simulink model "test_asus"  (R2015a)
settings: Solver=ode3  StartTime=0.0  StopTime=5.0  RelTol=1e-3
values from neighbouring files (symbols this model uses):
  cx = 159.5    [Initialize_camera.m]
  cy = 119.5    [Initialize_camera.m]
  focal = 525/2    (= 262.5)    [Initialize_camera.m]
  interval = 5    [Initialize_camera.m]
settings Model: SimulationMode=external  ExtModeTrigDuration=100  Creator=sarag  LastModifiedBy=Amanda
settings OptimizationCC: OptimizeModelRefInitCode=on  LifeSpan=1  MaxStackSize=64
settings DebuggingCC: UnderspecifiedInitializationDetection=Classic  MergeDetectMultiDrivingBlocksExec=none
settings HardwareCC: ProdLargestAtomicInteger=Long  ProdLargestAtomicFloat=Double  ProdEndianess=LittleEndian  ProdHWDeviceType=ARM Compatible->ARM Cortex
settings RTWCC: SystemTargetFile=realtime.tlc  GenerateMakefile=off  TemplateMakefile=realtime.tmf  Description=Run on Target Hardware  RTWVerbose=off  Toolchain=Linaro Toolchain v4.8
settings ERTTargetCC: CombineOutputUpdateFcns=off  ExtModeMexArgs='192.168.7.2' 0 17725  ERTSrcFileBannerTemplate=realtime_code_template.cgt  ERTHdrFileBannerTemplate=realtime_code_template.cgt  ERTDataSrcFileTemplate=realtime_code_template.cgt  ERTDataHdrFileTemplate=realtime_code_template.cgt  ERTCustomFileTemplate=realtime_file_process.tlc

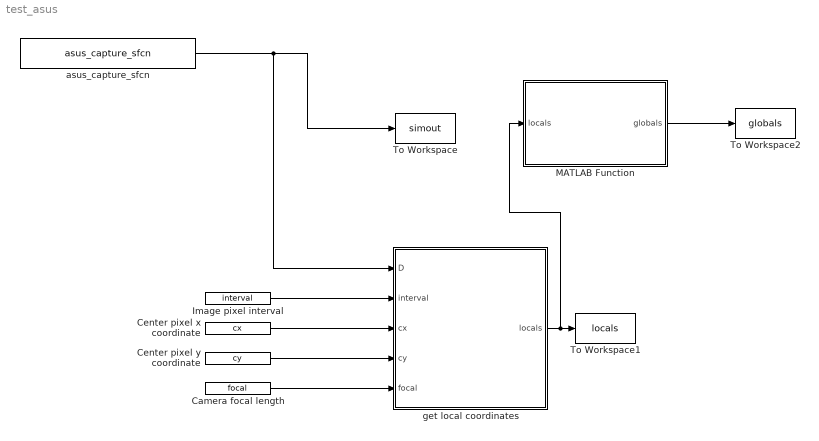
== system test_asus ==
  Camera focal length : Constant  Value=focal  SampleTime=-1
  Center pixel x coordinate : Constant  Value=cx  SampleTime=-1
  Center pixel y coordinate : Constant  Value=cy  SampleTime=-1
  Image pixel interval : Constant  Value=interval  SampleTime=-1
  MATLAB Function : MATLAB Function  TreatAsAtomicUnit=on
  To Workspace : ToWorkspace  VariableName=simout  SampleTime=-1
  To Workspace1 : ToWorkspace  VariableName=locals  SampleTime=-1
  To Workspace2 : ToWorkspace  VariableName=globals  SampleTime=-1
  asus_capture_sfcn : S-Function  FunctionName=asus_capture_sfcn  Parameters=SampleTime  mask(Legacy Function){SFunctionSpec=asusCapture(uint16 y1[240][320]), SampleTime=-1, ShowSpec=on}
      mask prompts: SampleTime "Sample time (-1 for inherited):"; ShowSpec "Display function specification"
      mask help:
      | This block allows you to call the legacy functions specified by the following Legacy Code Tool definition:
      | def.SFunctionName = 'asus_capture_sfcn';
      | def.OutputFcnSpec = 'asusCapture(uint16 y1[240][320])';
      | def.StartFcnSpec = 'asusInit()';
      | def.TerminateFcnSpec = 'asusTerminate()';
      | def.HeaderFiles = {'asus_capture.h', 'NI.h', 'wrapper.h'};
      | def.SourceFiles = {'wrapper.c'};
      | def.TargetLibFiles = {'libNI.so'};
      | def.IncPaths = {'.\include'};
      | def.SrcPaths = {'.\src'};
      | def.SampleTime = 'parameterized';
      | def.Options.isMacro = true;
      | def.Options.useTlcWithAccel = false;
      mask Help: <p>This block was generated automatically by the Legacy Code Tool. For detailed help on this tool, call<a href="matlab:legacy_code('help')"> legacy_code('help')</a>.</p>
      mask Callback ShowSpec:
      | if strcmp(get_param(gcbh, 'ShowSpec'), 'on')
      |   set_param(gcbh, 'MaskDisplay', sprintf('fprintf(''%s'');', get_param(gcbh, 'SFunctionSpec')));
      | else
      |   set_param(gcbh, 'MaskDisplay', sprintf('fprintf(''%s'');', get_param(gcbh, 'FunctionName')));
      | end
      mask Display: fprintf('asusCapture(uint16 y1[240][320])');
  get local coordinates : MATLAB Function  TreatAsAtomicUnit=on
  wires:
  Image pixel interval/1 -> get local coordinates/2(interval)
  Center pixel x coordinate/1 -> get local coordinates/3(cx)
  Center pixel y coordinate/1 -> get local coordinates/4(cy)
  Camera focal length/1 -> get local coordinates/5(focal)
  asus_capture_sfcn/1 -> get local coordinates/1(D), To Workspace/1
  get local coordinates/1(locals) -> MATLAB Function/1(locals), To Workspace1/1
  MATLAB Function/1(globals) -> To Workspace2/1

== matlab function test_asus/MATLAB Function ==
  data: locals input; globals output
function globals   = getGlobalCoordinates(locals)
B = zeros(size(locals));
Bt = zeros(4,length(locals));
globals = zeros(size(locals));


dt = zeros(4,4);

x = zeros(1, 3072);
y = zeros(1, 3072);
z = zeros(1, 3072);

R = eye(3);
    t = zeros(3,1);

    dt = [R t; 0 0 0 1];
    % Transformed cloud
    Bt = dt * [locals; ones(1,size(locals,2))];
    globals = Bt(1:3, :);  
    
end

== matlab function test_asus/get local coordinates ==
  data: D input; locals output; interval input; cx input; cy input; focal input
function locals = getLocalCoordinates(D, interval, cx,cy, focal)
%#codegen
a = 1;
x = zeros(1, 3072); %12288
y = zeros(1, 3072);
z = zeros(1, 3072);
D = double(D)/1000;  %is in mm

[r,c] = size(D);
for i = 1:interval:r                                         %row -> i,  col->j
    for j = 1:interval:c
        zz = D(i,j);
        if (zz > 0)    
            % Pinhole camera model
            Bx = ((j - cx)*zz/focal);
            By = ((i - cy)*zz/focal); 
            Bz = zz;   

            globals = [Bx;By;Bz;1];                 % To place coordinates in the world frame

            x(a) = globals(1);
            y(a) = globals(2);
            z(a) = globals(3);
            a = a+1;          
            
        end
    end
end    
 locals = [x; y; z];
end
